simulink model "Model"  (Simulink 8.5)
settings: Solver=ode45  StartTime=0.0  StopTime=.001  RelTol=1e-3
values from neighbouring files (symbols this model uses):
  C = 10e-6    (= 1e-05)    [configuration.m]
  K = R2/(R2+R1)    (= 0.666666666667)    [configuration.m]
  R1 = 10    [configuration.m]
  R2 = 20    [configuration.m]
  T = R1*R2*C/(R1+R2)    (= 6.66666666667e-05)    [configuration.m]
settings Model: Creator=Estudiantes  LastModifiedBy=Daniel Santos
settings DebuggingCC: SolverPrmCheckMsg=warning  FcnCallInpInsideContextMsg=EnableAllAsWarning
settings GRTTargetCC: CombineOutputUpdateFcns=on  GRTInterface=off

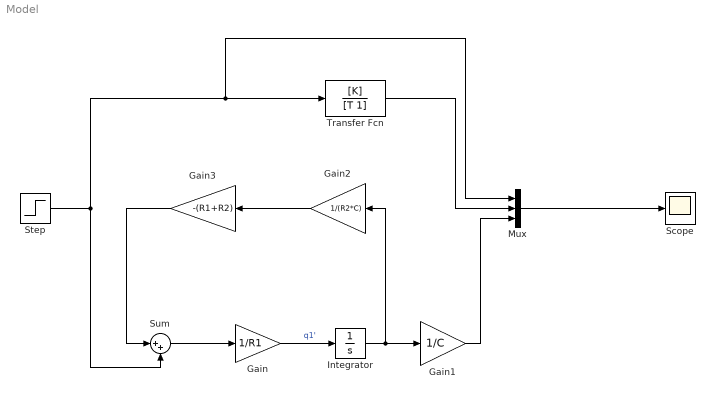
== system Model ==
  Gain : Gain  Gain=1/R1
  Gain1 : Gain  Gain=1/C
  Gain2 : Gain  Gain=1/(R2*C)
  Gain3 : Gain  Gain=-(R1+R2)
  Integrator : Integrator
  Mux : Mux  Inputs=3
  Scope : Scope
      settings: YMin=0  YMax=1
  Step : Step  Time=0  SampleTime=0
  Sum : Sum  Inputs=|++
  Transfer Fcn : TransferFcn  Numerator=[K]  Denominator=[T 1]
  wires:
  Step/1 -> Transfer Fcn/1, Mux/1, Sum/2
  Transfer Fcn/1 -> Mux/2
  Mux/1 -> Scope/1
  Sum/1 -> Gain/1
  Gain/1 -> Integrator/1  "q1'"
  Integrator/1 -> Gain1/1, Gain2/1
  Gain1/1 -> Mux/3
  Gain2/1 -> Gain3/1
  Gain3/1 -> Sum/1
